simulink model "FactorialLoopFunc"  (R2018b)
settings: Solver=FixedStepDiscrete  StartTime=0.0  StopTime=10.0  RelTol=1e-3
settings Model: Creator=Ahmed Soliman  LastModifiedBy=Ahmed Soliman
settings OptimizationCC: DefaultParameterBehavior=Inlined  EnhancedBackFolding=on  PassReuseOutputArgsAs=Individual arguments  OptimizeBlockOrder=speed  DifferentSizesBufferReuse=on  OptimizationCustomize=off
settings DebuggingCC: UnderspecifiedInitializationDetection=Classic  MergeDetectMultiDrivingBlocksExec=none  ParameterTunabilityLossMsg=error
settings ModelReferenceCC: PropagateSignalLabelsOutOfModel=off
settings SFSimCC: MATLABDynamicMemAlloc=off
settings RTWCC: SystemTargetFile=ert.tlc  GenCodeOnly=on  TemplateMakefile=ert_default_tmf  GenerateReport=on  IncludeHyperlinkInReport=on  LaunchReport=on  GenerateTraceInfo=on  GenerateTraceReport=on  GenerateTraceReportSl=on  GenerateTraceReportSf=on  GenerateTraceReportEml=on
settings CodeAppCC: ForceParamTrailComments=on  IgnoreCustomStorageClasses=off  OperatorAnnotations=on  SimulinkDataObjDesc=on  SFDataObjDesc=on  InsertBlockDesc=on
settings ERTTargetCC: TargetLangStandard=C99 (ISO)  GenerateSampleERTMain=on  InlinedParameterPlacement=NonHierarchical  ERTCustomFileTemplate=example_file_process.tlc

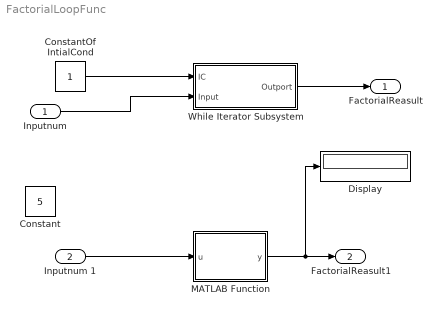
== system FactorialLoopFunc ==
  "Inputnum " : Inport
  Inputnum 1 : Inport  Port=2  OutDataTypeStr=uint16
  Constant : Constant  Value=5
  ConstantOf IntialCond : Constant  OutDataTypeStr=uint16
  Display : Display
  MATLAB Function : MATLAB Function  TreatAsAtomicUnit=on
  While Iterator Subsystem : Subsystem  TreatAsAtomicUnit=on
  FactorialReasult : Outport
  FactorialReasult1 : Outport  Port=2
  wires:
  ConstantOf IntialCond/1 -> While Iterator Subsystem/1(IC)
  While Iterator Subsystem/1(Outport) -> FactorialReasult/1
  "Inputnum "/1 -> While Iterator Subsystem/2(Input)
  MATLAB Function/1(y) -> Display/1, FactorialReasult1/1
  Inputnum 1/1 -> MATLAB Function/1(u)

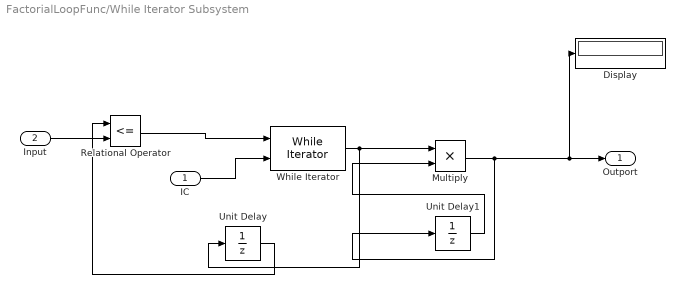
== system FactorialLoopFunc/While Iterator Subsystem ==
  IC : Inport  OutDataTypeStr=uint16
  Input : Inport  Port=2
  Display : Display
  Multiply : Product
  Relational Operator : RelationalOperator  Operator=<=  OutDataTypeStr=boolean  RndMeth=Simplest
  Unit Delay : UnitDelay  InitialCondition=1  SampleTime=-1
  Unit Delay1 : UnitDelay  InitialCondition=1  SampleTime=-1
  While Iterator : WhileIterator  ResetStates=reset  ShowIterationPort=on  OutputDataType=double
  Outport : Outport
  wires:
  IC/1 -> While Iterator/2
  Input/1 -> Relational Operator/2
  Unit Delay/1 -> Relational Operator/1
  While Iterator/1 -> Multiply/1, Unit Delay/1
  Relational Operator/1 -> While Iterator/1
  Multiply/1 -> Unit Delay1/1, Display/1, Outport/1
  Unit Delay1/1 -> Multiply/2

== matlab function FactorialLoopFunc/MATLAB Function ==
  data: u input; y output
function y = fcn(u)
n = 1;
y = 1;
while n <= u
    y = y * n;
    n = n + 1;
end
end
